simulink model "zad9_repr_graf_niel_i_zlin_dyn_mod_dyskretny"  (R2014b)
settings: Solver=ode45  StartTime=0.0  StopTime=1000.0  RelTol=1e-3
values from neighbouring files (symbols this model uses):
  a1 = 0.39    [dane_poczatkowe.mat]
  a2 = 0.45    [dane_poczatkowe.mat]
  a3 = -2.91    [dane_poczatkowe.mat]
  a4 = 0.25    [dane_poczatkowe.mat]
  K = 3.5    [dane_poczatkowe.mat]
  T1 = 5    [dane_poczatkowe.mat]
  T2 = 9    [dane_poczatkowe.mat]
  Tp = 0.1    [dane_poczatkowe.mat]
  x1 = 0    [dane_poczatkowe.mat]
  x2 = 0    [dane_poczatkowe.mat]
undefined symbols (not defined in the file or in its folder): U
settings Model: Creator=Konrad  LastModifiedBy=Konrad

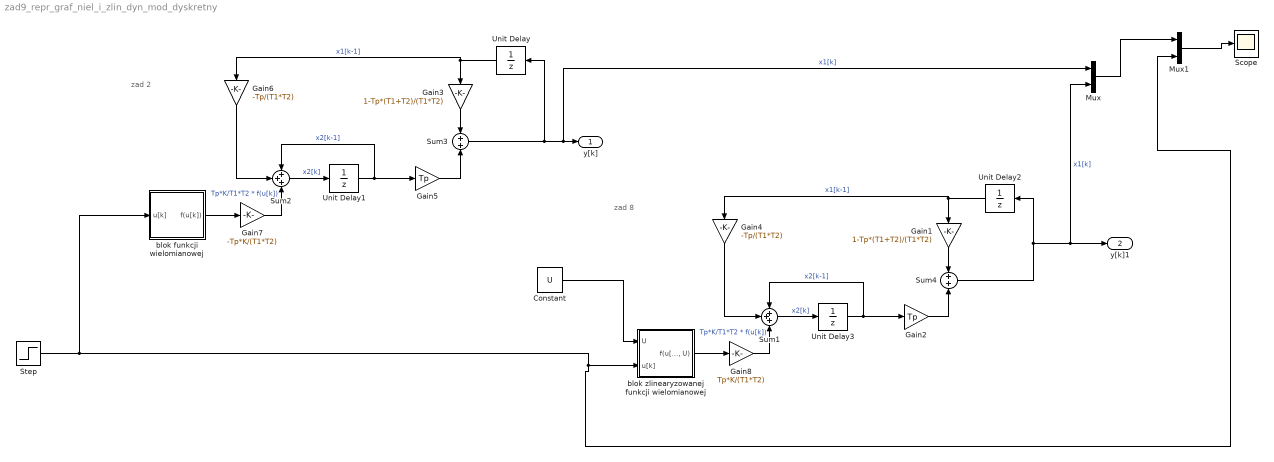
== system zad9_repr_graf_niel_i_zlin_dyn_mod_dyskretny ==
  note: zad 8
  note: zad 2
  Constant : Constant  Value=U
  Gain1 : Gain  Gain=1-Tp*(T1+T2)/(T1*T2)
  Gain2 : Gain  Gain=Tp
  Gain3 : Gain  Gain=1-Tp*(T1+T2)/(T1*T2)
  Gain4 : Gain  Gain=-Tp/(T1*T2)
  Gain5 : Gain  Gain=Tp
  Gain6 : Gain  Gain=-Tp/(T1*T2)
  Gain7 : Gain  Gain=-Tp*K/(T1*T2)
  Gain8 : Gain  Gain=Tp*K/(T1*T2)
  Mux : Mux  Inputs=2
  Mux1 : Mux  Inputs=2
  Scope : Scope
  Step : Step  SampleTime=0
  Sum1 : Sum  Inputs=+++
  Sum2 : Sum  Inputs=+++
  Sum3 : Sum  Inputs=+|+
  Sum4 : Sum  Inputs=+|+
  Unit Delay : UnitDelay  InitialCondition=x1  SampleTime=Tp
  Unit Delay1 : UnitDelay  InitialCondition=x2  SampleTime=Tp
  Unit Delay2 : UnitDelay  InitialCondition=x1  SampleTime=Tp
  Unit Delay3 : UnitDelay  InitialCondition=x2  SampleTime=Tp
  blok funkcji wielomianowej : Subsystem
  blok zlinearyzowanej funkcji wielomianowej : Subsystem
  y[k] : Outport
  y[k]1 : Outport  Port=2
  wires:
  Sum3/1 -> Unit Delay/1, Mux/1, y[k]/1  "x1[k]"
  Unit Delay/1 -> Gain6/1, Gain3/1  "x1[k-1]"
  Gain3/1 -> Sum3/1
  Unit Delay1/1 -> Gain5/1, Sum2/1  "x2[k-1]"
  Gain5/1 -> Sum3/2
  Sum2/1 -> Unit Delay1/1  "x2[k]"
  Gain6/1 -> Sum2/2
  Step/1 -> blok funkcji wielomianowej/1(u[k]), blok zlinearyzowanej funkcji wielomianowej/2(u[k]), Mux1/2
  blok funkcji wielomianowej/1(f(u[k])) -> Gain7/1
  Gain7/1 -> Sum2/3  "Tp*K/T1*T2 * f(u[k])"
  Sum4/1 -> Unit Delay2/1, Mux/2, y[k]1/1  "x1[k]"
  Unit Delay2/1 -> Gain4/1, Gain1/1  "x1[k-1]"
  Gain1/1 -> Sum4/1
  Unit Delay3/1 -> Gain2/1, Sum1/1  "x2[k-1]"
  Gain2/1 -> Sum4/2
  Sum1/1 -> Unit Delay3/1  "x2[k]"
  Gain4/1 -> Sum1/2
  Gain8/1 -> Sum1/3  "Tp*K/T1*T2 * f(u[k])"
  Constant/1 -> blok zlinearyzowanej funkcji wielomianowej/1(U)
  blok zlinearyzowanej funkcji wielomianowej/1("f(u[k], U)") -> Gain8/1
  Mux1/1 -> Scope/1
  Mux/1 -> Mux1/1

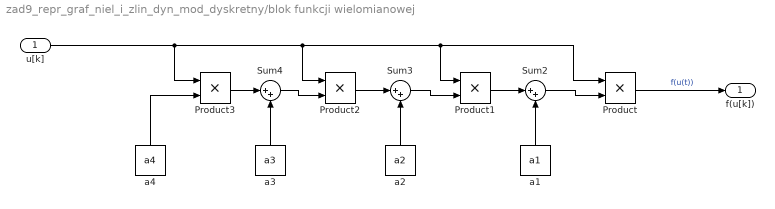
== system zad9_repr_graf_niel_i_zlin_dyn_mod_dyskretny/blok funkcji wielomianowej ==
  u[k] : Inport
  Product{,1..3} (4 alike) : Product
  Sum2 : Sum  Inputs=|++
  Sum3 : Sum  Inputs=|++
  Sum4 : Sum  Inputs=|++
  a1 : Constant  Value=a1
  a2 : Constant  Value=a2
  a3 : Constant  Value=a3
  a4 : Constant  Value=a4
  f(u[k]) : Outport
  wires:
  u[k]/1 -> Product/1, Product1/1, Product2/1, Product3/1
  Product1/1 -> Sum2/1
  Product2/1 -> Sum3/1
  Sum2/1 -> Product/2
  Product/1 -> f(u[k])/1  "f(u(t))"
  Product3/1 -> Sum4/1
  a1/1 -> Sum2/2
  a2/1 -> Sum3/2
  Sum3/1 -> Product1/2
  a3/1 -> Sum4/2
  Sum4/1 -> Product2/2
  a4/1 -> Product3/2

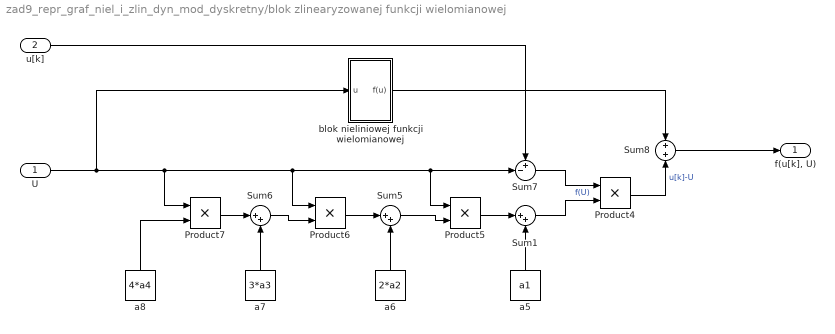
== system zad9_repr_graf_niel_i_zlin_dyn_mod_dyskretny/blok zlinearyzowanej funkcji wielomianowej ==
  U : Inport
  u[k] : Inport  Port=2
  Product{4..7} (4 alike) : Product
  Sum1 : Sum  Inputs=|++
  Sum5 : Sum  Inputs=|++
  Sum6 : Sum  Inputs=|++
  Sum7 : Sum  Inputs=+-|
  Sum8 : Sum
  a5 : Constant  Value=a1
  a6 : Constant  Value=2*a2
  a7 : Constant  Value=3*a3
  a8 : Constant  Value=4*a4
  blok nieliniowej funkcji wielomianowej : Subsystem
  "f(u[k], U)" : Outport
  wires:
  U/1 -> blok nieliniowej funkcji wielomianowej/1(u), Product5/1, Sum7/2, Product6/1, Product7/1
  Product5/1 -> Sum1/1
  Product6/1 -> Sum5/1
  Product7/1 -> Sum6/1
  a5/1 -> Sum1/2
  a6/1 -> Sum5/2
  Sum5/1 -> Product5/2
  a7/1 -> Sum6/2
  Sum6/1 -> Product6/2
  a8/1 -> Product7/2
  Sum1/1 -> Product4/2  "f(U)"
  Sum7/1 -> Product4/1
  u[k]/1 -> Sum7/1
  Product4/1 -> Sum8/2  "u[k]-U"
  Sum8/1 -> "f(u[k], U)"/1
  blok nieliniowej funkcji wielomianowej/1(f(u)) -> Sum8/1

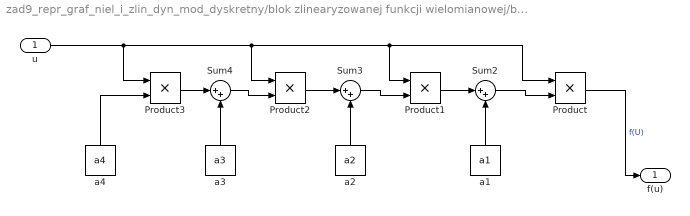
== system zad9_repr_graf_niel_i_zlin_dyn_mod_dyskretny/blok zlinearyzowanej funkcji wielomianowej/blok nieliniowej funkcji wielomianowej ==
  u : Inport
  Product{,1..3} (4 alike) : Product
  Sum2 : Sum  Inputs=|++
  Sum3 : Sum  Inputs=|++
  Sum4 : Sum  Inputs=|++
  a1 : Constant  Value=a1
  a2 : Constant  Value=a2
  a3 : Constant  Value=a3
  a4 : Constant  Value=a4
  f(u) : Outport
  wires:
  u/1 -> Product/1, Product1/1, Product2/1, Product3/1
  Product2/1 -> Sum3/1
  Sum2/1 -> Product/2
  Product/1 -> f(u)/1  "f(U)"
  Product3/1 -> Sum4/1
  a1/1 -> Sum2/2
  a2/1 -> Sum3/2
  Sum3/1 -> Product1/2
  Sum4/1 -> Product2/2
  a3/1 -> Sum4/2
  a4/1 -> Product3/2
  Product1/1 -> Sum2/1
